simulink model "untitled"  (R2020b)
settings: Solver=VariableStepAuto  StartTime=0.0  StopTime=5  MaxStep=1e-6  RelTol=1e-3
libraries: dspsrcs4 x1
settings Model: Creator=pawel  LastModifiedBy=pawel

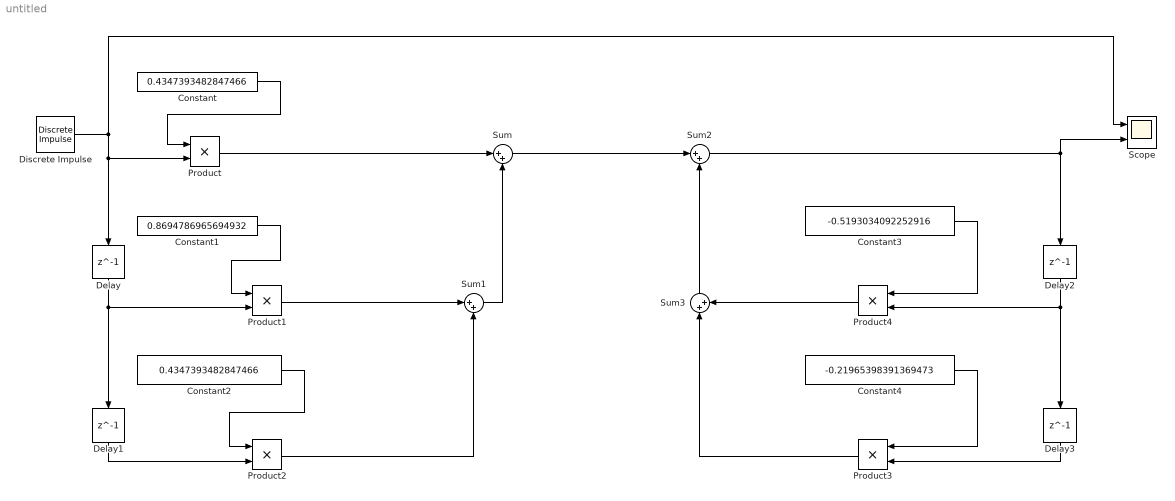
== system untitled ==
  Constant : Constant  Value=0.4347393482847466
  Constant1 : Constant  Value=0.8694786965694932
  Constant2 : Constant  Value=0.4347393482847466
  Constant3 : Constant  Value=-0.5193034092252916
  Constant4 : Constant  Value=-0.21965398391369473
  Delay{,1..3} (4 alike) : Delay  DelayLength=1  InitialCondition=0
  Discrete Impulse : dspsrcs4/Discrete  Impulse  Delay=5000  SampleTime=1/5000  FrameSample=1  OutputFrames=off  dataType=double  isSigned=on  wordLen=16  udDataType=sfix(16)  fracBitsMode=Best precision  numFracBits=15  OutDataTypeStr=double  LastOutDataTypeStr=double
  Product{,1..4} (5 alike) : Product
  Scope : Scope  NumInputPorts=2
  Sum{,1..3} (4 alike) : Sum  Inputs=|++
  wires:
  Sum2/1 -> Scope/2, Delay2/1
  Sum3/1 -> Sum2/2
  Constant2/1 -> Product2/1
  Product/1 -> Sum/1
  Product2/1 -> Sum1/2
  Sum/1 -> Sum2/1
  Constant/1 -> Product/1
  Delay3/1 -> Product3/2
  Constant1/1 -> Product1/1
  Product4/1 -> Sum3/2
  Delay/1 -> Delay1/1, Product1/2
  Discrete Impulse/1 -> Delay/1, Product/2, Scope/1
  Product1/1 -> Sum1/1
  Delay1/1 -> Product2/2
  Product3/1 -> Sum3/1
  Constant4/1 -> Product3/1
  Sum1/1 -> Sum/2
  Constant3/1 -> Product4/1
  Delay2/1 -> Product4/2, Delay3/1
